simulink model "opencircuit"  (R2022b)
settings: Solver=ode45  StartTime=0.0  StopTime=0.01  MaxStep=1e-8  RelTol=1e-3
undefined symbols (not defined in the file or in its folder): plecs
libraries: plecslib_extras2 x1, simulink x1
settings Model: Creator=qawse  LastModifiedBy=qawse
settings DataIOCC: ReturnWorkspaceOutputs=off

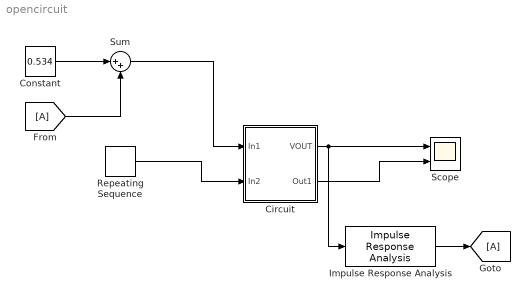
== system opencircuit ==
  Circuit : Subsystem  LoadFcn=plecs('sl', 200);  InitFcn=plecs('sl', 214);  StartFcn=plecs('sl', 208);  StopFcn=plecs('sl', 209);  mask(PlecsCircuit){PLECSData=<binary blob, 3100 chars, not shown>}
      mask prompts: PLECSData "PLECS Data (Do not delete or modify!)"
      mask init:
      | % PLACE CUSTOM INITIALIZATIONS ABOVE
      | % DO NOT REMOVE
      | plecs('sl', 215);
      | % DO NOT REMOVE
      settings: CopyFcn=plecs('sl', 203);  DeleteFcn=plecs('sl', 205);  UndoDeleteFcn=plecs('sl', 206);  PreSaveFcn=plecs('sl', 211);  PostSaveFcn=plecs('sl', 201);  NameChangeFcn=plecs('sl', 210);  DestroyFcn=plecs('sl', 207);  PreCopyFcn=plecs('sl', 216);  OpenFcn=plecs('sl', 202);  ErrorFcn=plerrorfcn
      mask Help: web(['file:///' fullfile(plecsdoc, 'creatingacircuit.html')])
      mask Display: disp('PLECS\nCircuit')
  Constant : Constant  Value=0.534
  From : From
  Goto : Goto
  Impulse Response Analysis : plecslib_extras2/Analysis Tools/Impulse Response Analysis  FreqRange=[100 500000]  FreqScale=logarithmic  NPoints=1000  Perturbation=1e-3  Compensation=discrete pulse  TimeSpan=1e-6  TStart=0  MaxIter=20  Tolerance=1e-6  Display=iteration  HideScopes=on  HiddenStates=error  OutputName=T  BodePlot=on  JPert=1e-4  NInitCycles=0
      settings: SourceProductName=PLECS Extras
  Repeating Sequence : simulink/Sources/Repeating Sequence  rep_seq_t=[0 2e-6]  rep_seq_y=[0 3]
  Scope : Scope  NumInputPorts=2
  Sum : Sum  Inputs=|++
  wires:
  Repeating Sequence/1 -> Circuit/2(In2)
  Circuit/1(VOUT) -> Scope/1, Impulse Response Analysis/1
  Circuit/2(Out1) -> Scope/2
  Constant/1 -> Sum/1
  From/1 -> Sum/2
  Sum/1 -> Circuit/1(In1)
  Impulse Response Analysis/1 -> Goto/1

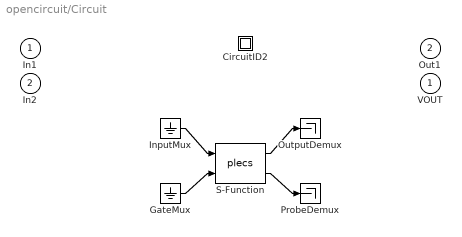
== system opencircuit/Circuit ==
  In1 : Inport  PortDimensions=1
  In2 : Inport  Port=2  PortDimensions=1
  " CircuitID2 " : Subsystem
  " GateMux " : Ground
  " InputMux " : Ground
  " OutputDemux " : Terminator
  " ProbeDemux " : Terminator
  " S-Function " : S-Function  FunctionName=plecs  SFunctionDeploymentMode=off  EnableBusSupport=off
  VOUT : Outport  PortDimensions=1
  Out1 : Outport  Port=2  PortDimensions=1
  wires:
  " InputMux "/1 -> " S-Function "/1
  " GateMux "/1 -> " S-Function "/2
  " S-Function "/1 -> " OutputDemux "/1
  " S-Function "/2 -> " ProbeDemux "/1

== system opencircuit/Circuit/ CircuitID2  ==
